simulink model "MCC"  (R2024b)
settings: Solver=ode15s  StartTime=0.0  StopTime=0.2  RelTol=1e-3
InitFcn:
  | parameters
StartFcn:
  | parameters
values from neighbouring files (symbols this model uses):
  b = 3.5077e-6    (= 3.5077e-06)    [parameters.m]
  Cr = 0    [parametretp3.m]
  J = 3.2284e-6    (= 3.2284e-06)    [parameters.m]    (also in parametretp3.m = 0.2)
  K = 0.9    [parametretp3.m]
  L = 2.75e-6    (= 2.75e-06)    [parameters.m]    (also in parametretp3.m = 0.012161)
  R = 4    [parameters.m]    (also in parametretp3.m = 0.895)
undefined symbols (not defined in the file or in its folder): U
settings Model: Creator=E306-PC5  LastModifiedBy=E306-PC5

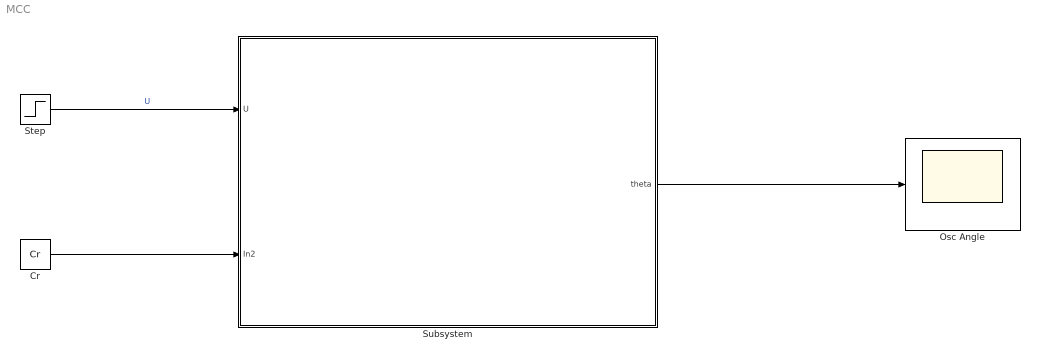
== system MCC ==
  Cr : Constant  Value=Cr
  Osc Angle : Scope
  Step : Step  Time=0.1  After=U  SampleTime=0
  Subsystem : Subsystem
  wires:
  Step/1 -> Subsystem/1(U)  "U"
  Cr/1 -> Subsystem/2(In2)
  Subsystem/1(theta) -> Osc Angle/1

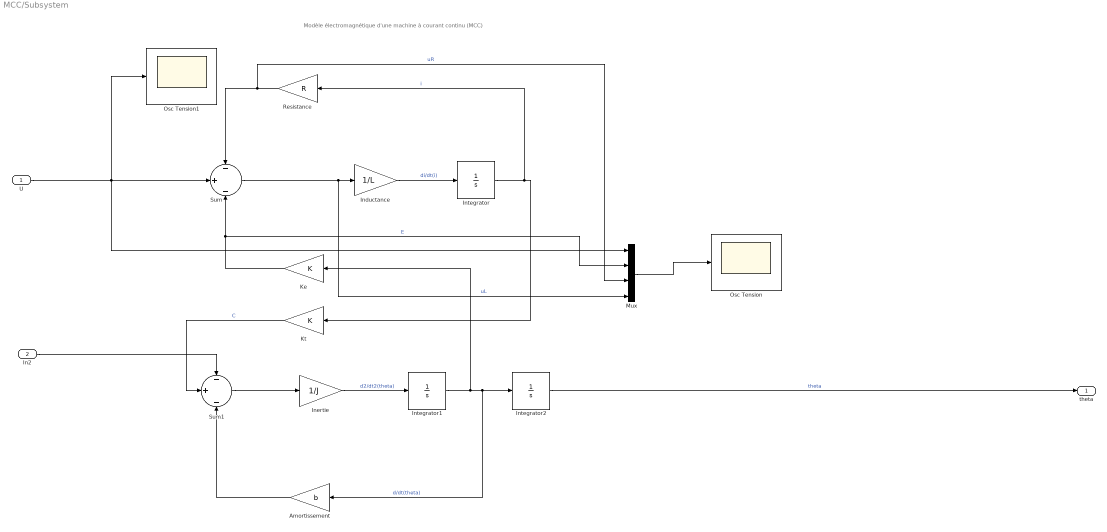
== system MCC/Subsystem ==
  note: Modèle électromagnétique d'une machine à courant continu (MCC)
  U : Inport
  In2 : Inport  Port=2
  Amortissement : Gain  Gain=b
  Inductance : Gain  Gain=1/L
  Inertie : Gain  Gain=1/J
  Integrator : Integrator
  Integrator1 : Integrator
  Integrator2 : Integrator
  Ke : Gain  Gain=K
  Kt : Gain  Gain=K
  Mux : Mux
  Osc Tension : Scope
  Osc Tension1 : Scope
  Resistance : Gain  Gain=R
  Sum : Sum  Inputs=-|+|-
  Sum1 : Sum  Inputs=-|+|-
  theta : Outport
  wires:
  In2/1 -> Sum1/1
  Resistance/1 -> Mux/3, Sum/1  "uR"
  Ke/1 -> Sum/3, Mux/2  "E"
  Inductance/1 -> Integrator/1  "di/dt(i)"
  Sum/1 -> Mux/4, Inductance/1  "uL"
  Integrator/1 -> Resistance/1, Kt/1  "i"
  Integrator1/1 -> Ke/1, Amortissement/1, Integrator2/1  "d/dt(theta)"
  Sum1/1 -> Inertie/1
  Inertie/1 -> Integrator1/1  "d2/dt2(theta)"
  U/1 -> Osc Tension1/1, Mux/1, Sum/2
  Amortissement/1 -> Sum1/3
  Kt/1 -> Sum1/2  "C"
  Integrator2/1 -> theta/1  "theta"
  Mux/1 -> Osc Tension/1
